simulink model "simulation_path_following"  (R2020b)
settings: Solver=VariableStepAuto  StartTime=0.0  StopTime=50  FixedStep=0.0001  RelTol=1e-2
values from neighbouring files (symbols this model uses):
  controlleur = struct('k1',0.01,                       'kc',1.0                       )    [generateContolleur.m]    (also in run_path_following.m = generateContolleur())
  initial_state = [p_initial; v_initial; q_initial; omega_initial]    [run_path_following.m]
  p1 = [0;0;0]    [run_path_following.m]
  p2 = [1000; 1000; 0]    [run_path_following.m]
libraries: simulink_extras x3, sharedtransform x1
settings Model: Creator=florian  LastModifiedBy=florian

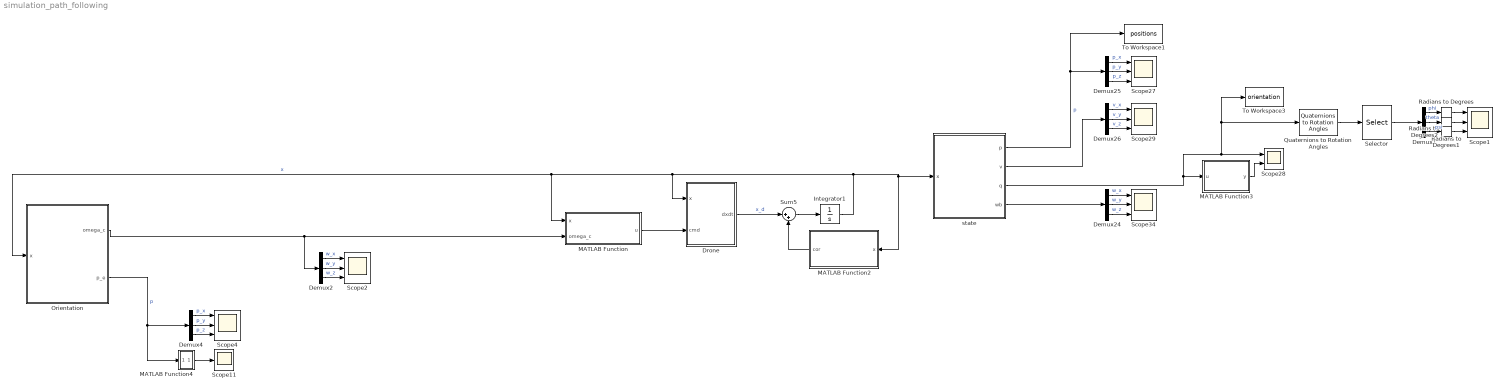
== system simulation_path_following ==
  Demux{1..2,4,24..26} (6 alike) : Demux  Outputs=3
  Drone : MATLAB Function  TreatAsAtomicUnit=on
  Integrator1 : Integrator  InitialCondition=initial_state
  MATLAB Function : MATLAB Function  TreatAsAtomicUnit=on
  MATLAB Function2 : MATLAB Function  TreatAsAtomicUnit=on
  MATLAB Function3 : MATLAB Function  TreatAsAtomicUnit=on
  MATLAB Function4 : MATLAB Function  TreatAsAtomicUnit=on
  Orientation : MATLAB Function  TreatAsAtomicUnit=on
  Quaternions to Rotation Angles : sharedtransform/Quaternions to Rotation Angles  rotationOrder=ZXY  aMode=aMode
      settings: SourceProductBaseCode=AE,PW,MT,UV,VE,VP
  Radians to Degrees : simulink_extras/Transformations/Radians to Degrees
  Radians to Degrees1 : simulink_extras/Transformations/Radians to Degrees
  Radians to Degrees2 : simulink_extras/Transformations/Radians to Degrees
  Scope{1..2,4,27,29,34} (6 alike) : Scope  NumInputPorts=3
  Scope11 : Scope
  Scope28 : Scope  NumInputPorts=2
  Selector : Selector  InputPortWidth=3  IndexOptions=Index vector (dialog)  Indices=[2 3 1]  OutputSizes=1
  Sum5 : Sum  Inputs=|++
  To Workspace1 : ToWorkspace  VariableName=positions  SampleTime=-1
  To Workspace3 : ToWorkspace  VariableName=orientation  SampleTime=-1
  state : MATLAB Function  TreatAsAtomicUnit=on
  wires:
  Demux24/1 -> Scope34/1  "w_x"
  MATLAB Function3/1(y) -> Scope28/2
  Drone/1(dxdt) -> Sum5/1  "x_d"
  Demux24/2 -> Scope34/2  "w_y"
  Demux25/2 -> Scope27/2  "p_y"
  Integrator1/1 -> MATLAB Function/1(x), Orientation/1(x), Drone/1(x), MATLAB Function2/1(x), state/1(x)  "x"
  state/3(q) -> Scope28/1, To Workspace3/1, Quaternions to Rotation Angles/1, MATLAB Function3/1(u)
  Sum5/1 -> Integrator1/1
  MATLAB Function2/1(cor) -> Sum5/2
  Demux26/3 -> Scope29/3  "v_z"
  Demux26/2 -> Scope29/2  "v_y"
  Demux25/1 -> Scope27/1  "p_x"
  Demux25/3 -> Scope27/3  "p_z"
  state/1(p) -> To Workspace1/1, Demux25/1  "p"
  Demux24/3 -> Scope34/3  "w_z"
  Demux26/1 -> Scope29/1  "v_x"
  Quaternions to Rotation Angles/1 -> Selector/1
  Selector/1 -> Demux1/1
  Orientation/1(omega_c) -> MATLAB Function/2(omega_c), Demux2/1
  state/2(v) -> Demux26/1
  state/4(wb) -> Demux24/1
  Demux2/1 -> Scope2/1  "w_x"
  Demux2/3 -> Scope2/3  "w_z"
  Demux2/2 -> Scope2/2  "w_y"
  Demux4/3 -> Scope4/3  "p_z"
  Demux4/2 -> Scope4/2  "p_y"
  Demux4/1 -> Scope4/1  "p_x"
  Orientation/2(p_e) -> MATLAB Function4/1(u), Demux4/1  "p"
  MATLAB Function4/1(y) -> Scope11/1
  Demux1/1 -> Radians to Degrees/1  "phi"
  Radians to Degrees/1 -> Scope1/1
  Demux1/2 -> Radians to Degrees1/1  "theta"
  Radians to Degrees1/1 -> Scope1/2
  Demux1/3 -> Radians to Degrees2/1  "psi"
  Radians to Degrees2/1 -> Scope1/3
  MATLAB Function/1(u) -> Drone/2(cmd)

== matlab function simulation_path_following/MATLAB Function ==
  data: x input; u output; omega_c input
function u = fcn(x, omega_c)

% p = x(1:3);
% v = x(4:6);
% q  = x(7:10);
wb = x(11:13);

J = diag([0.007018 0.002785 0.00606]);

u = cross(wb, J*wb) + 1* (omega_c - wb);

== matlab function simulation_path_following/Drone ==
  data: x input; cmd input size=3; dxdt output
function dxdt  = drone(x, cmd)



%% state demultiplexing
% p = x(1:3);
v = x(4:6);
q  = x(7:10);
wb = x(11:13);

% position
u = quadprod(quadprod(q, [0;v]),quadconj(q)); 
dpdt = u(2:4);

% kinematics
dvdt =  [0;0;0]; 


%% quaternion derivative
% eta = q(1);
% eps = q(2:4);
% 
% dqdt = (1/2)*[-eps'; eta*eye(3) + skew_sym(eps)]*wb;
dqdt = quadprod(1/2*q, [0;wb]);

%% angular velocity derivative
% kinematics
% dwdt = 1*(omega_c - wb);
J = diag([0.007018 0.002785 0.00606]);
J_inv = inv(J);
dwdt = -J_inv* cross(wb, J*wb) + J_inv*cmd;

%% derivative multiplexing
dxdt = [dpdt; dvdt; dqdt; dwdt] ;

== matlab function simulation_path_following/MATLAB Function4 ==
  data: u input; y output
function y = fcn(u)
%#codegen

y = norm(u);

== matlab function simulation_path_following/Orientation ==
  data: x input; omega_c output; p1 parameter; p2 parameter; controlleur parameter; p_e output
function [omega_c, p_e]= orientation(x, p1, p2, controlleur)
%#codegen
p = x(1:3);
% v = x(4:6);
q  = x(7:10);
% w = x(11:13);

u_p = (p2-p1)/norm(p2-p1);

khi_p = atan2(u_p(1), u_p(2));
gamma_p = -atan2(u_p(3), sqrt(u_p(1)^2 + u_p(2)^2));

q_p_khi = [cos(khi_p/2); 0; 0; sin(khi_p/2)];
q_p_gamma = [cos(gamma_p/2); 0; sin(gamma_p/2); 0];

q_n_p = quadprod(q_p_khi, q_p_gamma);

p_e = ((p-p1)'*u_p)*u_p + p1-p;

khi_c = atan2(p_e(2), p_e(1));
gamma_c = -atan2(p_e(3), sqrt(p_e(1)^2 + p_e(2)^2));


q_c_khi = [cos(khi_c/2); 0; 0; sin(khi_c/2)];
q_c_gamma = [cos(gamma_c/2); 0; sin(gamma_c/2); 0];

q_n_c = quadprod(q_c_khi, q_c_gamma);

q_n_d = (q_n_p - q_n_c)*exp(-controlleur.k1*norm(p_e)) + q_n_c;
%q_n_d = q_n_p ;
q_e = quadprod(quadconj(q_n_d), q);

omega_c = -controlleur.kc*q_e(1)*q_e(2:4);

== matlab function simulation_path_following/MATLAB Function2 ==
  data: x input; cor output
function cor  = fcn(x)
%#codegen
q  = x(7:10);
n = norm(q);
mismatch = 1-n;
cor = [0;0;0; 0;0;0; mismatch*q; 0;0;0];

== matlab function simulation_path_following/MATLAB Function3 ==
  data: u input; y output
function y = fcn(u)
%#codegen

y = norm(u);

== matlab function simulation_path_following/state ==
  data: x input; p output; v output; q output; wb output
function [p, v,q, wb] = demux(x)
%#codegen

p = x(1:3);
v = x(4:6);
q  = x(7:10);
wb = x(11:13);
